simulink model "test"  (R2015b)
settings: Solver=VariableStepAuto  StartTime=0.0  StopTime=200  RelTol=1e-3
settings Model: Creator=rajiv  LastModifiedBy=rajiv

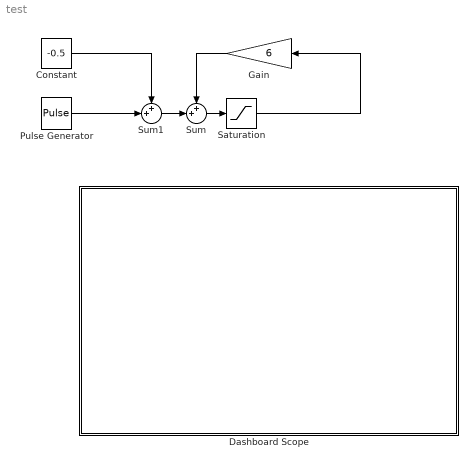
== system test ==
  Constant : Constant  Value=-0.5
  Dashboard Scope : Subsystem  DialogController=hmiCreateDDGDialog  IsWebBlock=on  mask(MWDashboardBlock){webBlockId=6df1c8a0-6efe-4b6a-a3ab-6f26fd3792df, webBlockType=sdiscope, ShowInitialText=on, HMISrcModelName=test}
      mask prompts: webBlockId "WebBlock Id"; webBlockType "WebBlock Type"; HMISrcModelName "Source Model"
      mask Help: helpview([docroot '/mapfiles/simulink.map'], 'hmi_scope')
      mask Display:
      | if strcmp(get_param(bdroot(gcb),'BlockDiagramType'), 'library')
      |     image([(matlabroot) '/toolbox/simulink/hmi/icons/DashboardScope.png']);
      | end
  Gain : Gain  Gain=6
  Pulse Generator : DiscretePulseGenerator  PulseType=Time based  Amplitude=.1  Period=100  PulseWidth=50
  Saturation : Saturate  UpperLimit=1  LowerLimit=-1
  Sum : Sum  Inputs=++|
  Sum1 : Sum  Inputs=++|
  wires:
  Saturation/1 -> Gain/1
  Gain/1 -> Sum/1
  Constant/1 -> Sum1/1
  Sum/1 -> Saturation/1
  Pulse Generator/1 -> Sum1/2
  Sum1/1 -> Sum/2

== system test/Dashboard Scope ==
